simulink model "freq_eval"  (Simulink 3.00)
libraries: mathlib x17, analoglib x4, arclib x1

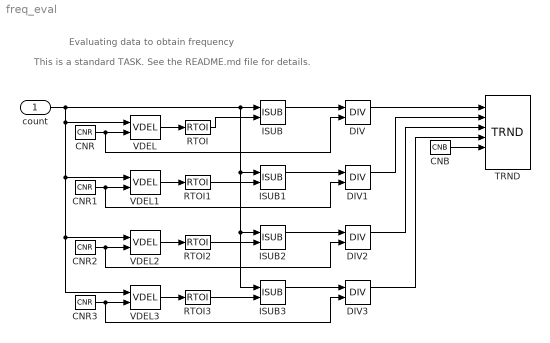
== system freq_eval ==
  note: Evaluating data to obtain frequency
  note: This is a standard TASK. See the README.md file for details.
  count : Inport  Port=1
  CNB : mathlib/CNB  YCN=on
  CNR : mathlib/CNR  ycn=0.5
  CNR1 : mathlib/CNR  ycn=1
  CNR2 : mathlib/CNR  ycn=2
  CNR3 : mathlib/CNR  ycn=5
  DIV{,1..3} (4 alike) : mathlib/DIV  yerr=-1
  ISUB{,1..3} (4 alike) : mathlib/ISUB  vtype=4: Long  SAT=off
  RTOI{,1..3} (4 alike) : mathlib/RTOI
  TRND : arclib/TRND  n=4  l=10000  btype=8: Double  ptype1=1: Store  ptype2=1: Store  ptype3=1: Store  ptype4=1: Store  pfac=1  afac=0  arc=0  id=1  Title=Frequency of the pulses  timesrc=1
  VDEL{,1..3} (4 alike) : analoglib/VDEL  y0=0  nmax=100
  wires:
  CNB/1 -> TRND/5
  CNR/1 -> DIV/2, VDEL/2
  CNR1/1 -> DIV1/2, VDEL1/2
  CNR2/1 -> DIV2/2, VDEL2/2
  CNR3/1 -> DIV3/2, VDEL3/2
  DIV/1 -> TRND/1
  DIV1/1 -> TRND/2
  DIV2/1 -> TRND/3
  DIV3/1 -> TRND/4
  ISUB/1 -> DIV/1
  ISUB1/1 -> DIV1/1
  ISUB2/1 -> DIV2/1
  ISUB3/1 -> DIV3/1
  RTOI/1 -> ISUB/2
  RTOI1/1 -> ISUB1/2
  RTOI2/1 -> ISUB2/2
  RTOI3/1 -> ISUB3/2
  VDEL/1 -> RTOI/1
  VDEL1/1 -> RTOI1/1
  VDEL2/1 -> RTOI2/1
  VDEL3/1 -> RTOI3/1
  count/1 -> ISUB1/1, ISUB2/1, ISUB3/1, ISUB/1, VDEL/1, VDEL1/1, VDEL2/1, VDEL3/1
